simulink model "zad_6_sch"  (R2022b)
settings: Solver=FixedStepAuto  StartTime=0.0  StopTime=1  FixedStep=0.0001  RelTol=1e-3
undefined symbols (not defined in the file): A, B, C, Kx, u0, x1, x2, x3, xd
settings Model: Creator=AgraWoodAdmin  LastModifiedBy=MPatr

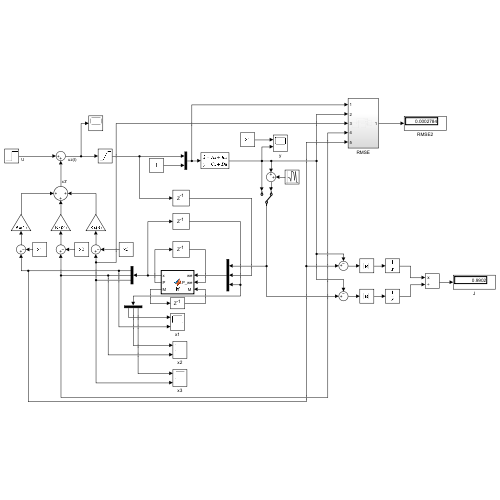
[thumbnail: Simulink's stored preview of the top-level diagram]
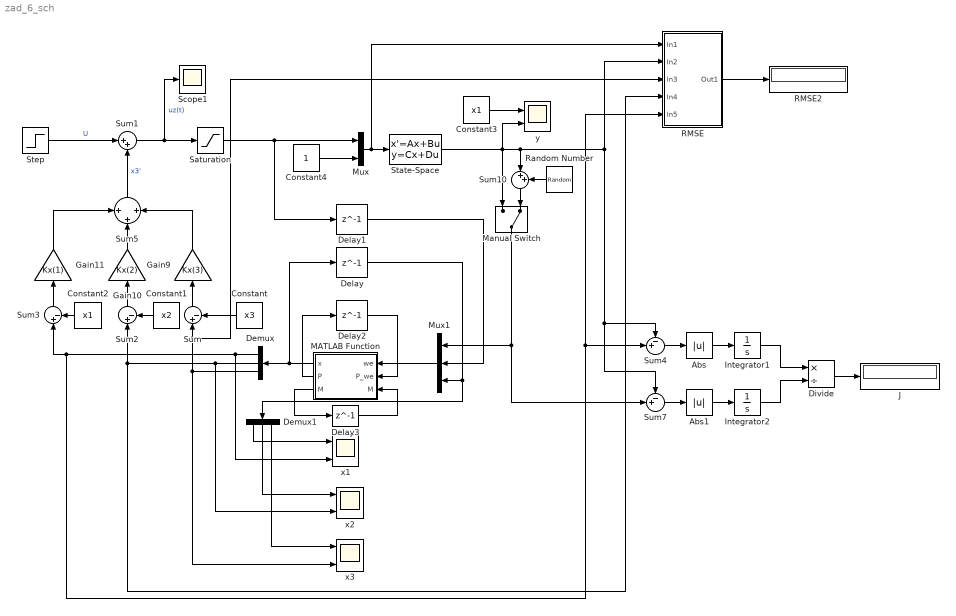
== system zad_6_sch ==
  Abs : Abs  SaturateOnIntegerOverflow=off
  Abs1 : Abs  SaturateOnIntegerOverflow=off
  Constant : Constant  Value=x3
  Constant1 : Constant  Value=x2
  Constant2 : Constant  Value=x1
  Constant3 : Constant  Value=x1
  Constant4 : Constant
  Delay : Delay  DelayLength=1  InitialCondition=[xd; 0; 0]
  Delay1 : Delay  DelayLength=1  InitialCondition=0
  Delay2 : Delay  DelayLength=1  InitialCondition=[0 0 0; 0 0 0; 0 0 0]
  Delay3 : Delay  DelayLength=1  InitialCondition=0
  Demux : Demux  Outputs=3
  Demux1 : Demux  Outputs=3
  Divide : Product  Inputs=*/
  Gain10 : Gain  Gain=Kx(2)
  Gain11 : Gain  Gain=Kx(1)
  Gain9 : Gain  Gain=Kx(3)
  Integrator1 : Integrator
  Integrator2 : Integrator
  J : Display
  MATLAB Function : MATLAB Function  TreatAsAtomicUnit=on
  Manual Switch : ManualSwitch  CurrentSetting=0
  Mux : Mux  Inputs=2
  Mux1 : Mux  Inputs=3
  RMSE : Subsystem
  RMSE2 : Display
  Random Number : RandomNumber  Variance=.0000001
  Saturation : Saturate  UpperLimit=1  LowerLimit=0
  Scope1 : Scope
  State-Space : StateSpace  A=A  B=B  C=C  D=[0 0]  InitialCondition=[xd; 0; 0]
  Step : Step  Time=0  After=u0  SampleTime=0
  Sum : Sum  Inputs=|+-
  Sum1 : Sum  Inputs=|++
  Sum10 : Sum  Inputs=|++
  Sum2 : Sum  Inputs=|+-
  Sum3 : Sum  Inputs=|+-
  Sum4 : Sum  Inputs=-+|
  Sum5 : Sum  Inputs=+|+|+
  Sum7 : Sum  Inputs=-+|
  x1 : Scope  NumInputPorts=2
  x2 : Scope  NumInputPorts=2
  x3 : Scope  NumInputPorts=2
  y : Scope  NumInputPorts=2
  wires:
  Demux/3 -> x3/2, RMSE/3(In3), Sum/1
  Gain9/1 -> Sum5/3
  Sum1/1 -> Saturation/1, Scope1/1  "uz(t)"
  Demux/2 -> Sum2/1, RMSE/4(In4), x2/2
  Sum5/1 -> Sum1/2  "x3'"
  Gain10/1 -> Sum5/2
  Sum10/1 -> Manual Switch/2
  Step/1 -> Sum1/1  "U"
  Gain11/1 -> Sum5/1
  Mux/1 -> RMSE/1(In1), State-Space/1
  State-Space/1 -> RMSE/2(In2), Sum7/1, Sum4/1, Sum10/1, y/2, Manual Switch/1
  Random Number/1 -> Sum10/2
  Constant4/1 -> Mux/2
  Delay/1 -> Demux1/1, Mux1/3
  Mux1/1 -> MATLAB Function/1(we)
  MATLAB Function/1(x) -> Demux/1, Delay/1
  Manual Switch/1 -> Sum7/2, Mux1/1
  Delay1/1 -> Mux1/2
  Saturation/1 -> Mux/1, Delay1/1
  Sum/1 -> Gain9/1
  Constant/1 -> Sum/2
  Sum2/1 -> Gain10/1
  Sum3/1 -> Gain11/1
  Constant1/1 -> Sum2/2
  Constant2/1 -> Sum3/2
  Constant3/1 -> y/1
  MATLAB Function/2(P) -> Delay2/1
  Delay2/1 -> MATLAB Function/2(P_we)
  Demux1/3 -> x3/1
  Demux1/2 -> x2/1
  Demux1/1 -> x1/1
  Demux/1 -> x1/2, RMSE/5(In5), Sum4/2, Sum3/1
  MATLAB Function/3(M) -> Delay3/1
  Delay3/1 -> MATLAB Function/3("M ")
  Integrator1/1 -> Divide/1
  Integrator2/1 -> Divide/2
  Sum4/1 -> Abs/1
  Abs/1 -> Integrator1/1
  Sum7/1 -> Abs1/1
  Abs1/1 -> Integrator2/1
  Divide/1 -> J/1
  RMSE/1(Out1) -> RMSE2/1

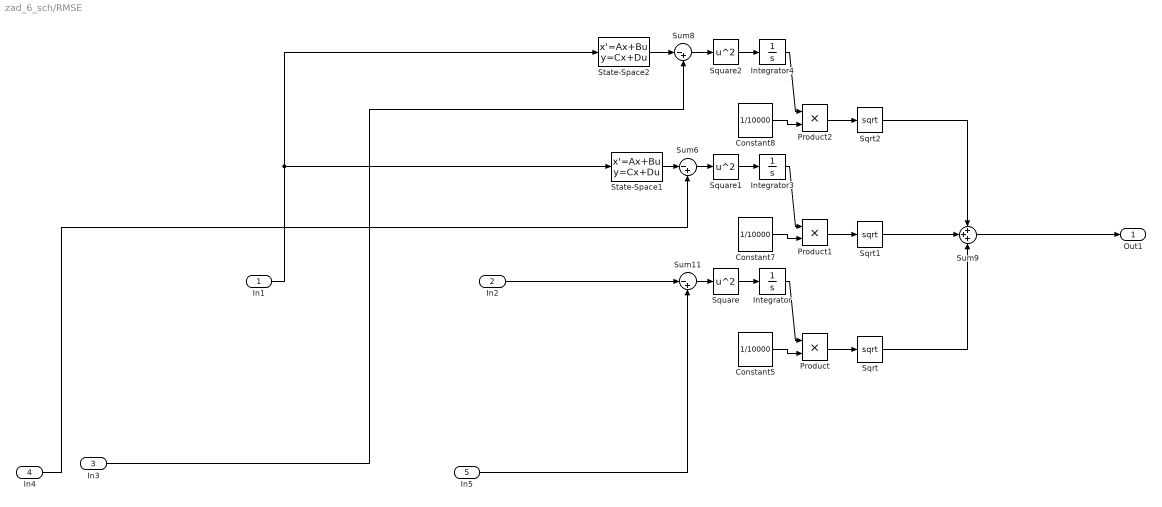
== system zad_6_sch/RMSE ==
  In1 : Inport
  In2 : Inport  Port=2
  In3 : Inport  Port=3
  In4 : Inport  Port=4
  In5 : Inport  Port=5
  Constant5 : Constant  Value=1/10000
  Constant7 : Constant  Value=1/10000
  Constant8 : Constant  Value=1/10000
  Integrator : Integrator
  Integrator3 : Integrator
  Integrator4 : Integrator
  Product : Product
  Product1 : Product
  Product2 : Product
  Sqrt : Sqrt
  Sqrt1 : Sqrt
  Sqrt2 : Sqrt
  Square : Math  Operator=square
  Square1 : Math  Operator=square
  Square2 : Math  Operator=square
  State-Space1 : StateSpace  A=A  B=B  C=[0 1 0]  D=[0 0]  InitialCondition=[xd; 0; 0]
  State-Space2 : StateSpace  A=A  B=B  C=[0 0 1]  D=[0 0]  InitialCondition=[xd; 0; 0]
  Sum11 : Sum  Inputs=|-+
  Sum6 : Sum  Inputs=|-+
  Sum8 : Sum  Inputs=|-+
  Sum9 : Sum  Inputs=+++
  Out1 : Outport
  wires:
  Integrator4/1 -> Product2/1
  Product/1 -> Sqrt/1
  State-Space1/1 -> Sum6/1
  Square/1 -> Integrator/1
  Sqrt2/1 -> Sum9/1
  Constant8/1 -> Product2/2
  Product1/1 -> Sqrt1/1
  Square2/1 -> Integrator4/1
  Product2/1 -> Sqrt2/1
  Integrator3/1 -> Product1/1
  In5/1 -> Sum11/2
  Sum11/1 -> Square/1
  In2/1 -> Sum11/1
  Constant7/1 -> Product1/2
  Integrator/1 -> Product/1
  Constant5/1 -> Product/2
  In1/1 -> State-Space2/1, State-Space1/1
  Square1/1 -> Integrator3/1
  State-Space2/1 -> Sum8/1
  Sum6/1 -> Square1/1
  Sum8/1 -> Square2/1
  Sqrt1/1 -> Sum9/2
  Sqrt/1 -> Sum9/3
  In4/1 -> Sum6/2
  In3/1 -> Sum8/2
  Sum9/1 -> Out1/1

== matlab function zad_6_sch/MATLAB Function ==
  data: we input; x output; P output; P_we input; M input; M output
function [x, P, M]  = kf(we, P_we, M)
%% Odczyt wejsc
y = we(1);  % aktualny pomiar
u = we(2);  % aktualne wymuszenie
x1 = we(3:5);   % poprzedni wektor stanu

%% Parametry
m = .00575;
g = 9.81;
FemP1 = .017521;
FemP2 = .0058231;
f1 = .00014142;
f2 = .0045626;
ki = 2.5165;
ci = .0243 * sign(4-2);
d = .0792;
bd = .06;
xd = d-bd;
x10 = .008;
x20 = 0;
x30 = .75;
u10 = 1/ki*(x30-ci);

a21 = 1/(2*m)*x30^2*FemP1/FemP2^2*exp(-x10/FemP2); 
a23 = -1/(m)*x30*FemP1/FemP2*exp(-x10/FemP2); 
a31 = 1/f1*exp(x10/f2)*(ki*u10+ci-x30); 
a33 = -f2/f1*exp(x10/f2);
b31 = ki*f2/f1*exp(x10/f2);

% Do sprawdzenia zakłóceń wewnętrzynych
% A = [0 1 0; a21 0 a23; a31*1.01 0 a33*1.02];
A = [0 1 0; a21 0 a23; a31 0 a33];
B = [0 0; 0 g; b31 0];
C = [1 0 0];
D = 0;

%% Dyskretyzacja modelu metodą Eulera w przód(na podstawie instrukcji lab5)
Tp = 0.0001;
Ad = (eye(3)+A*Tp);
Bd = B*Tp;
Cd = C;
Dd = D;

%% Nastawy filtru
var_n = 0.001; % wariancja szumu pomiarowego
var_v = 0.1; % wariancje szumow wewnetrznych

Q = diag([var_v, var_v, var_v]);    % macierz kowariancji szumow wewnetrznych
R = diag(var_n);  	% macierz kowariancji szumow pomiarowych

%% Algorytm filtru Kalmana
% Etap predykcji
x_d = Ad*x1 + Bd*[u; 1];
P_d = Ad*P_we*Ad' + Q;

% Etap filtracji
K = P_d*Cd' * ((Cd*P_d*Cd' + R)^-1);
x_hat = x_d + K*(y - Cd*x_d);

% Przekazanie danych
x = x_hat;
P = (eye(3)-K*Cd)*P_d;
M = M + 1;
end
